simulink model "ODE_PENDULUM"  (R2019b)
settings: Solver=VariableStepAuto  StartTime=0.0  StopTime=30  RelTol=1e-3
values from neighbouring files (symbols this model uses):
  c = 0.2    [Wahadlo.m]
  g = 10    [Wahadlo.m]
  L = 1    [Wahadlo.m]
  m = 1    [Wahadlo.m]
settings Model: Creator=szymo  LastModifiedBy=szymo

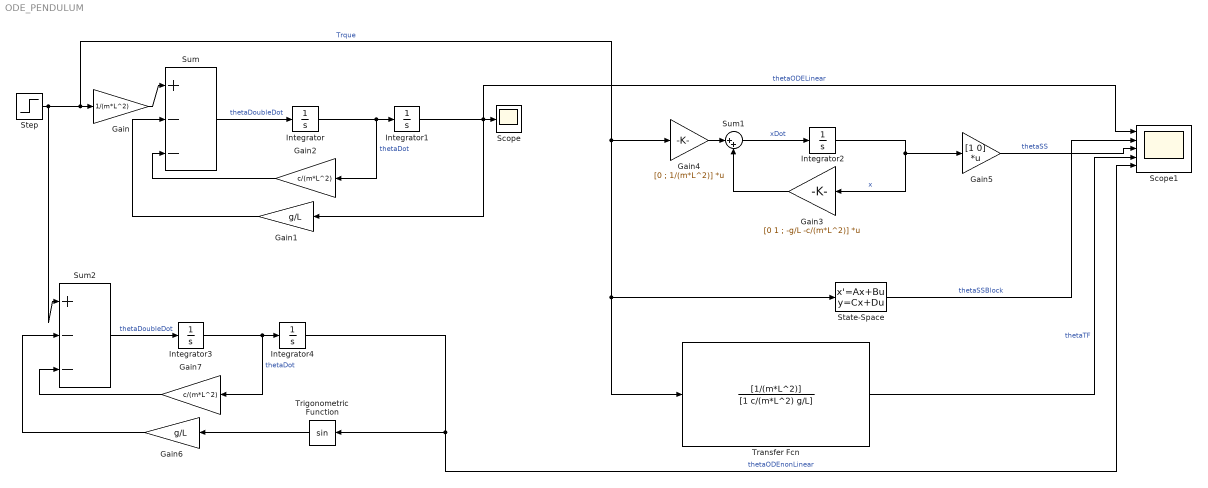
== system ODE_PENDULUM ==
  Gain : Gain  Gain=1/(m*L^2)
  Gain1 : Gain  Gain=g/L
  Gain2 : Gain  Gain=c/(m*L^2)
  Gain3 : Gain  Gain=[0 1 ; -g/L -c/(m*L^2)]  Multiplication=Matrix(K*u)
  Gain4 : Gain  Gain=[0 ; 1/(m*L^2)]  Multiplication=Matrix(K*u)
  Gain5 : Gain  Gain=[1 0]  Multiplication=Matrix(K*u)
  Gain6 : Gain  Gain=g/L
  Gain7 : Gain  Gain=c/(m*L^2)
  Integrator{,1..4} (5 alike) : Integrator
  Scope : Scope
  Scope1 : Scope  NumInputPorts=5
  State-Space : StateSpace  A=[0 1 ; -g/L -c/(m*L^2)]  B=[0 ; 1/(m*L^2)]  C=[1 0]  D=0  InitialCondition=0
  Step : Step  Time=3  SampleTime=0
  Sum : Sum  Inputs=|+--
  Sum1 : Sum  Inputs=|++
  Sum2 : Sum  Inputs=|+--
  Transfer Fcn : TransferFcn  Numerator=[1/(m*L^2)]  Denominator=[1 c/(m*L^2) g/L]
  Trigonometric Function : Trigonometry
  wires:
  Integrator/1 -> Gain2/1, Integrator1/1  "thetaDot"
  Sum/1 -> Integrator/1  "thetaDoubleDot"
  Integrator1/1 -> Gain1/1, Scope1/1, Scope/1  "thetaODELinear"
  Gain/1 -> Sum/1
  Gain2/1 -> Sum/3
  Gain1/1 -> Sum/2
  Sum1/1 -> Integrator2/1  "xDot"
  Integrator2/1 -> Gain3/1, Gain5/1  "x"
  Gain3/1 -> Sum1/2
  Gain4/1 -> Sum1/1
  Step/1 -> Sum2/1, Transfer Fcn/1, State-Space/1, Gain4/1, Gain/1  "Trque"
  Gain5/1 -> Scope1/3  "thetaSS"
  State-Space/1 -> Scope1/2  "thetaSSBlock"
  Transfer Fcn/1 -> Scope1/4  "thetaTF"
  Gain6/1 -> Sum2/2
  Integrator3/1 -> Gain7/1, Integrator4/1  "thetaDot"
  Gain7/1 -> Sum2/3
  Sum2/1 -> Integrator3/1  "thetaDoubleDot"
  Integrator4/1 -> Scope1/5, Trigonometric Function/1  "thetaODEnonLinear"
  Trigonometric Function/1 -> Gain6/1
